simulink model "Demodulation_SNR_AWGN"  (R2023a)
settings: Solver=VariableStepAuto  StartTime=0.0  StopTime=10.0  RelTol=1e-3
libraries: commchan3 x1, commanapbnd3 x1
settings Model: Creator=Pedro  LastModifiedBy=Pedro

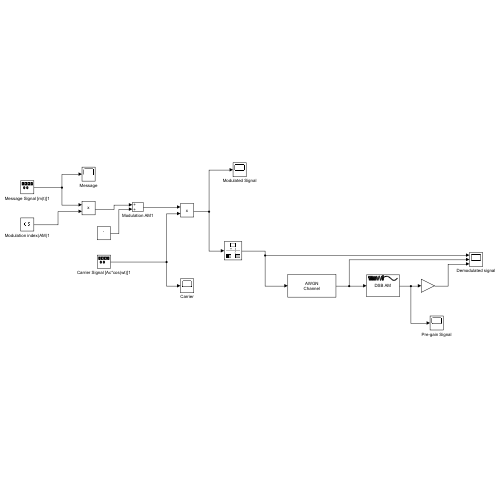
[thumbnail: Simulink's stored preview of the top-level diagram]
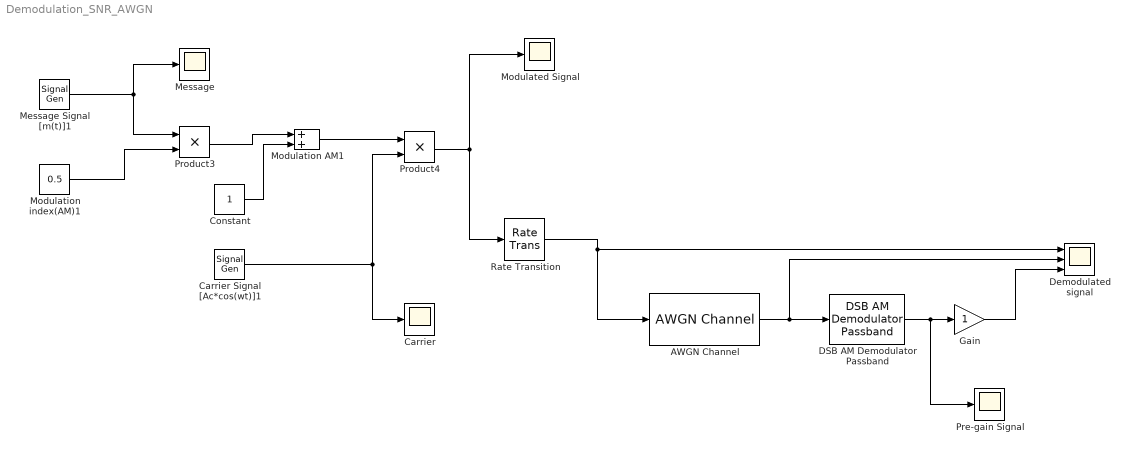
== system Demodulation_SNR_AWGN ==
  AWGN Channel : commchan3/AWGN Channel  LegacyMode=off  NoiseMethod="Signal to noise ratio  (SNR)"  noiseMode="Signal to noise ratio  (SNR)"  EbNo=10  EsNo=10  SNR=10  BitsPerSymbol=1  SignalPower=1  SamplesPerSymbol=1  SymbolPeriod=1  VarianceSource=Parameter  Variance=1  RandomStream=Global stream  Seed=67  SimulateUsing=Code generation
  Carrier : Scope
  Carrier Signal [Ac*cos(wt)]1 : SignalGenerator  Amplitude=2  Frequency=350
  Constant : Constant
  DSB AM Demodulator Passband : commanapbnd3/DSB AM Demodulator Passband  Fc=300  Ph=0  method=Butterworth  n=4  cf=300  Rp=0.1  Rs=50  Offset=1
  Demodulated signal : Scope  NumInputPorts=3
  Gain : Gain
  Message : Scope
  Message Signal [m(t)]1 : SignalGenerator  Frequency=150
  Modulated Signal : Scope
  Modulation AM1 : Sum
  Modulation index(AM)1 : Constant  Value=0.5
  Pre-gain Signal : Scope
  Product3 : Product
  Product4 : Product
  Rate Transition : RateTransition  OutPortSampleTime=0.001
  wires:
  Gain/1 -> Demodulated signal/3
  Modulation AM1/1 -> Product4/1
  Constant/1 -> Modulation AM1/2
  Product3/1 -> Modulation AM1/1
  Product4/1 -> Rate Transition/1, Modulated Signal/1
  Message Signal [m(t)]1/1 -> Product3/1, Message/1
  DSB AM Demodulator Passband/1 -> Pre-gain Signal/1, Gain/1
  AWGN Channel/1 -> Demodulated signal/2, DSB AM Demodulator Passband/1
  Modulation index(AM)1/1 -> Product3/2
  Rate Transition/1 -> AWGN Channel/1, Demodulated signal/1
  Carrier Signal [Ac*cos(wt)]1/1 -> Product4/2, Carrier/1
